simulink model "GasExample_V4S"  (R2025b)
settings: Solver=FixedStepAuto  StartTime=0.0  StopTime=1000  FixedStep=0.01  RelTol=1e-3
model workspace (MAT data in the model file):
  alpha = 20
libraries: Bibliothek_FHDO_V1 x23, BibFHDO x20, BibSpielo x11, simulink x9
(part 1 of 2)
settings Model: Creator=goessling  LastModifiedBy=henni

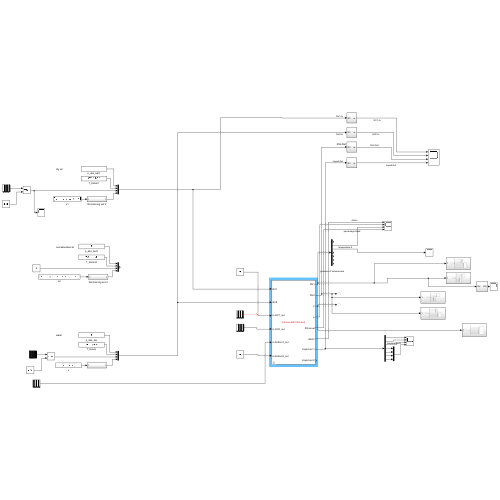
[thumbnail: Simulink's stored preview of the top-level diagram]
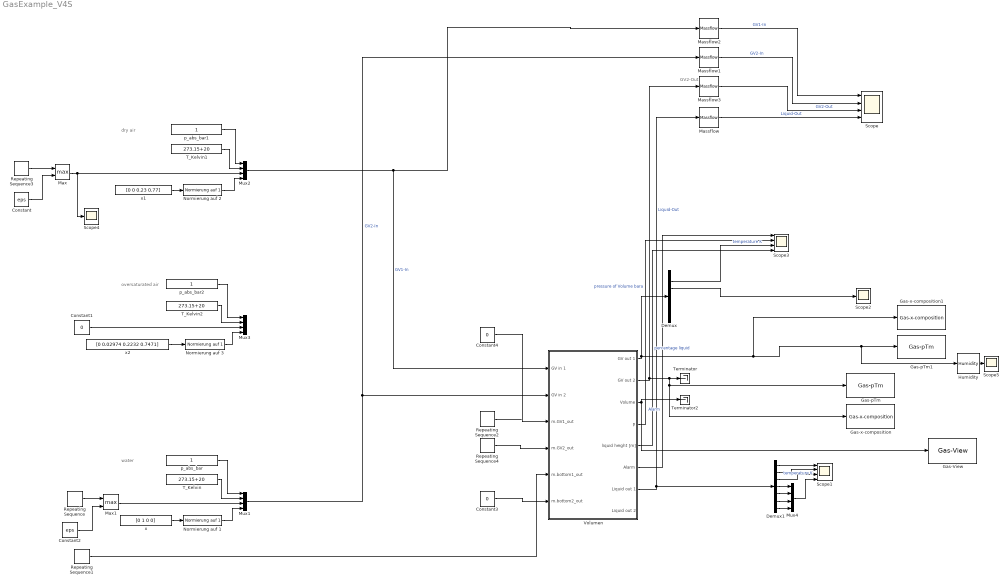
== system GasExample_V4S ==
  note: GV2-Out
  note: water
  note: dry air
  note: oversaturated air
  Constant : Constant  Value=eps
  Constant1 : Constant  Value=0
  Constant2 : Constant  Value=eps
  Constant3 : Constant  Value=0
  Constant4 : Constant  Value=0
  Demux : Demux  Outputs=7
  Demux1 : Demux  Outputs=7
  Gas-View : BibSpielo/Gas-View  SystemSampleTime=-1  VariantActivationTime=update diagram  EmptyChoice=off  PassThrough=off  PassThroughVariantControl=(default)  EmptyChoiceVariantControl=(default)  AllowFlexibleInterface=on  Latency=0  AutoFrameSizeCalculation=off
  Gas-pTm : BibSpielo/Gas-pTm  SystemSampleTime=-1  VariantActivationTime=update diagram  EmptyChoice=off  PassThrough=off  PassThroughVariantControl=(default)  EmptyChoiceVariantControl=(default)  AllowFlexibleInterface=on  Latency=0  AutoFrameSizeCalculation=off
  Gas-pTm1 : BibSpielo/Gas-pTm  SystemSampleTime=-1  VariantActivationTime=update diagram  EmptyChoice=off  PassThrough=off  PassThroughVariantControl=(default)  EmptyChoiceVariantControl=(default)  AllowFlexibleInterface=on  Latency=0  AutoFrameSizeCalculation=off
  Gas-x-composition : BibSpielo/Gas-x-composition  SystemSampleTime=-1  VariantActivationTime=update diagram  EmptyChoice=off  PassThrough=off  PassThroughVariantControl=(default)  EmptyChoiceVariantControl=(default)  AllowFlexibleInterface=on  Latency=0  AutoFrameSizeCalculation=off
  Gas-x-composition1 : BibFHDO/Gas-x-composition  SystemSampleTime=-1  VariantActivationTime=update diagram  EmptyChoice=off  PassThrough=off  PassThroughVariantControl=(default)  EmptyChoiceVariantControl=(default)  AllowFlexibleInterface=on  Latency=0  AutoFrameSizeCalculation=off
  Humidity : BibFHDO/Humidity  SystemSampleTime=-1  VariantActivationTime=update diagram  EmptyChoice=off  PassThrough=off  PassThroughVariantControl=(default)  EmptyChoiceVariantControl=(default)  AllowFlexibleInterface=on  Latency=0  AutoFrameSizeCalculation=off
  Massflow{,1..3} (4 alike) : BibSpielo/Massflow  SystemSampleTime=-1  VariantActivationTime=update diagram  EmptyChoice=off  PassThrough=off  PassThroughVariantControl=(default)  EmptyChoiceVariantControl=(default)  AllowFlexibleInterface=on  Latency=0  AutoFrameSizeCalculation=off
  Max : MinMax  Function=max  Inputs=2
  Max1 : MinMax  Function=max  Inputs=2
  Mux{1..4} (4 alike) : Mux
  Normierung auf 1 : BibSpielo/Normierung auf 1  SystemSampleTime=-1  VariantActivationTime=update diagram  EmptyChoice=off  PassThrough=off  PassThroughVariantControl=(default)  EmptyChoiceVariantControl=(default)  AllowFlexibleInterface=on  Latency=0  AutoFrameSizeCalculation=off
  Normierung auf 2 : BibSpielo/Normierung auf 1  SystemSampleTime=-1  VariantActivationTime=update diagram  EmptyChoice=off  PassThrough=off  PassThroughVariantControl=(default)  EmptyChoiceVariantControl=(default)  AllowFlexibleInterface=on  Latency=0  AutoFrameSizeCalculation=off
  Normierung auf 3 : BibSpielo/Normierung auf 1  SystemSampleTime=-1  VariantActivationTime=update diagram  EmptyChoice=off  PassThrough=off  PassThroughVariantControl=(default)  EmptyChoiceVariantControl=(default)  AllowFlexibleInterface=on  Latency=0  AutoFrameSizeCalculation=off
  Repeating Sequence : simulink/Sources/Repeating Sequence  rep_seq_t=[0 100 100.01 500 500.01 600 600.01 1000]  rep_seq_y=[1 1 0 0 1 1 0 0]*282.1778521
  Repeating Sequence1 : simulink/Sources/Repeating Sequence  rep_seq_t=[0 300 300.01 400 400.01 1000]  rep_seq_y=[0 0 1 1 0 0]*282.1778521
  Repeating Sequence2 : simulink/Sources/Repeating Sequence  rep_seq_t=[0 600 600.01 700 700.01 1000]  rep_seq_y=[0 0 1 1 0 0]*1
  Repeating Sequence3 : simulink/Sources/Repeating Sequence  rep_seq_t=[0 700 700.01 1000]  rep_seq_y=[0 0 1 1]*1
  Repeating Sequence4 : simulink/Sources/Repeating Sequence  rep_seq_t=[0 800 800.01 1000]  rep_seq_y=[0 0 1 1]*1
  Scope : Scope  NumInputPorts=4
      settings: ActiveDisplayYMinimum=-0.12499999999999972  ActiveDisplayYMaximum=1.125  DataLoggingVariableName=ScopeData5
  Scope1 : Scope  NumInputPorts=4
      settings: ActiveDisplayYMinimum=0.48520355295568851  ActiveDisplayYMaximum=7.0617394519702321
  Scope2 : Scope
      settings: ActiveDisplayYMinimum=-1.5770073931536848  ActiveDisplayYMaximum=1.2371934521588157  DataLoggingVariableName=ScopeData9
  Scope3 : Scope  NumInputPorts=4
      settings: ActiveDisplayYMinimum=-1  ActiveDisplayYMaximum=1
  Scope4 : Scope
      settings: ActiveDisplayYMinimum=-1  ActiveDisplayYMaximum=1  DataLoggingVariableName=ScopeData10
  Scope5 : Scope
      settings: ActiveDisplayYMinimum=-105.49899317481896  ActiveDisplayYMaximum=2813.8155771313386  DataLoggingVariableName=ScopeData3
  T_Kelvin : Constant  Value=273.15+20
  T_Kelvin1 : Constant  Value=273.15+20
  T_Kelvin2 : Constant  Value=273.15+20
  Terminator : Terminator
  Terminator2 : Terminator
  Volumen : Subsystem  mask{A=70685.83471/1000000, h=0.8, h_start=0.1, p_start=1, T_start=90, hum_start=50}
      mask prompts: A "Area [m^2]"; h "height [m]"; h_start "liquid level start [m]"; p_start "p [bar]"; T_start "T [°C]"; hum_start "Humidity [%]"
      mask Display:
      | color('red')
      | disp(['Volume with Fill-Level'])
      | 
      | color('black')
      | port_label('input', 1, 'GV1')
      | port_label('input', 2, 'GV2')
      | port_label('input', 3, 'm.GV1_out')
      | port_label('input', 4, 'm.GV2_out')
      | port_label('input', 5, 'm.bottom1_out')
      | port_label('input', 6, 'm.bottom2_out')
      | 
      | 
      | port_label('output', 1, 'GV1')
      | port_label('output', 2, 'GV2')
      | port_label('output', 3, 'V')
      | port_label('output', 4, 'p')
      | port_label('output', 5, 'Fill-Level')
      | port_label('output', 6, 'Alarm')
      | port_label('output', 7, 'Liquid out 1')
      | port_label('output', 8, 'Liquid out 2')
  p_abs_bar : Constant
  p_abs_bar1 : Constant
  p_abs_bar2 : Constant
  x : Constant  Value=[0 1 0 0]
  x1 : Constant  Value=[0 0 0.23 0.77]
  x2 : Constant  Value=[0 0.02974 0.2232 0.7471]
  wires:
  Volumen/3(Volume) -> Terminator2/1, Gas-View/1
  Volumen/4(p) -> Scope3/2  "pressure of Volume bara"
  Volumen/1(GV out 1) -> Gas-x-composition1/1, Humidity/1, Gas-pTm1/1, Demux/1
  Demux/2 -> Scope3/3  "temperature K"
  Volumen/5(liquid height [m]) -> Scope3/4  "percentage liquid"
  x/1 -> Normierung auf 1/1
  p_abs_bar/1 -> Mux1/1
  Mux1/1 -> Massflow1/1, Volumen/2(GV in 2)  "GV2-In"
  Repeating Sequence/1 -> Max1/1
  Normierung auf 1/1 -> Mux1/4
  T_Kelvin/1 -> Mux1/2
  T_Kelvin1/1 -> Mux2/2
  Normierung auf 2/1 -> Mux2/4
  Repeating Sequence3/1 -> Max/1
  p_abs_bar1/1 -> Mux2/1
  x1/1 -> Normierung auf 2/1
  T_Kelvin2/1 -> Mux3/2
  p_abs_bar2/1 -> Mux3/1
  x2/1 -> Normierung auf 3/1
  Normierung auf 3/1 -> Mux3/4
  Constant1/1 -> Mux3/3
  Mux2/1 -> Massflow2/1, Volumen/1(GV in 1)  "GV1-In"
  Volumen/6(Alarm) -> Scope3/1  "Alarm"
  Repeating Sequence1/1 -> Volumen/5(m.bottom1_out)
  Repeating Sequence4/1 -> Volumen/4(m.GV2_out)
  Constant3/1 -> Volumen/6(m.bottom2_out)
  Volumen/7(Liquid out 1) -> Massflow/1, Demux1/1  "Liquid-Out"
  Demux1/1 -> Scope1/1
  Demux1/2 -> Scope1/2  "temperature K"
  Demux1/3 -> Scope1/3
  Demux1/4 -> Mux4/1
  Demux1/5 -> Mux4/2
  Demux1/6 -> Mux4/3
  Demux1/7 -> Mux4/4
  Mux4/1 -> Scope1/4
  Repeating Sequence2/1 -> ?
  Constant/1 -> Max/2
  Max/1 -> Scope4/1, Mux2/3
  Constant2/1 -> Max1/2
  Max1/1 -> Mux1/3
  Constant4/1 -> Volumen/3(m.GV1_out)
  Demux/3 -> Scope2/1
  Volumen/2(GV out 2) -> Massflow3/1, Gas-pTm/1, Gas-x-composition/1, Terminator/1
  Massflow2/1 -> Scope/1  "GV1-In"
  Massflow1/1 -> Scope/2  "GV2-In"
  Massflow3/1 -> Scope/3  "GV2-Out"
  Massflow/1 -> Scope/4  "Liquid-Out"
  Humidity/1 -> Scope5/1

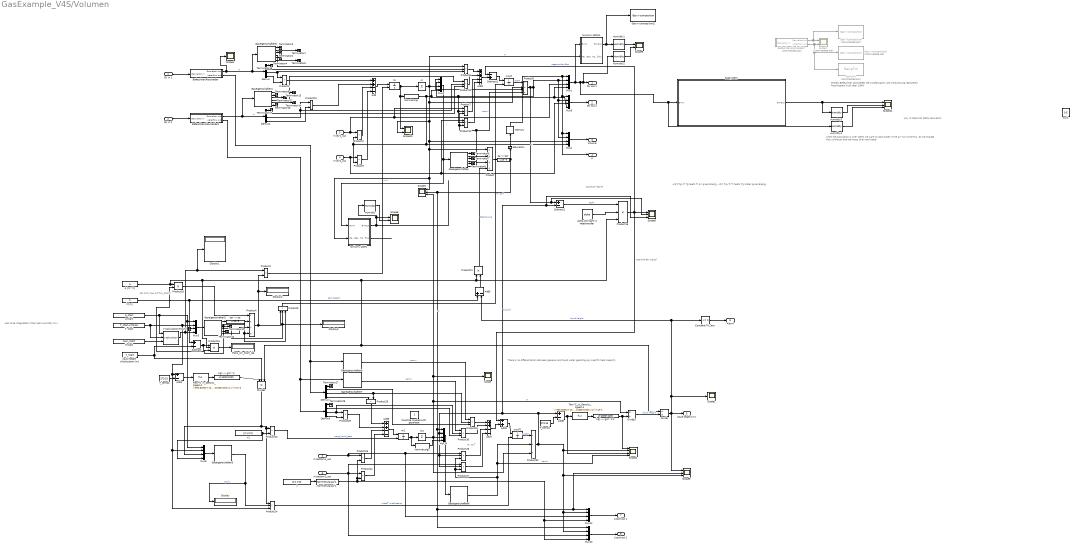
== system GasExample_V4S/Volumen ==
  note: why is there not 100% saturation
  note: when the saturation is over 100% we want to lose water in the air -[0 1 0 0]*mw.
      | So we change the x of the air and the mass of air and water
  note: Mittels Befeuchter Abscheider die Kondensation und Verdunstung realisieren
      | Feuchtigkeit nicht über 100%
  note: +Q=Tg>Tl Tg heats Tl Air gives Energy.
      | -Q= Tg<Tl Tl heats Tg Water gives Energy.
  note: 1st A*h, now A*(h-h_start)
  note: positive for Liquid
  note: Q=h*A*(Tg-Tl)
  note: There is no differentiation between gaseous and liquid water gearding e.g. spezific heat capacity
  note: m. cp T
  note: Has to be integrated in the mask Humidity to x
  GV in 1 : Inport
  GV in 2 : Inport  Port=2
  m.GV1_out : Inport  Port=3
  m.GV2_out : Inport  Port=4
  m.bottom1_out : Inport  Port=5
  m.bottom2_out : Inport  Port=6
  A [m^2] : Constant  Value=A
  Add : Sum  Inputs=++--
  Add1 : Sum  Inputs=++--  SampleTime=.01
  Add2 : Sum  Inputs=+-
  Add3 : Sum
  Add5 : Sum  Inputs=+-
  Add6 : Sum  Inputs=++--
  Add7 : Sum  Inputs=++--  SampleTime=.01
  Add8 : Sum  Inputs=+-
  Befeuchter/Abscheider : Subsystem
      mask Display:
      | color('red')
      | disp('No Oversaturation');
      | 
      | color('black')
      | port_label('output', 1, 'GV')
      | port_label('output', 2, 'm.')
      | port_label('input', 1, 'GV')
  Befeuchter/Abscheider1 : Subsystem
      mask Display:
      | color('red')
      | disp('No Oversaturation');
      | 
      | color('black')
      | port_label('output', 1, 'GV')
      | port_label('output', 2, 'm.')
      | port_label('input', 1, 'GV')
  Befeuchter/Abscheider2 : Subsystem  Commented=on
      mask Display:
      | color('red')
      | disp('No Oversaturation');
      | 
      | color('black')
      | port_label('output', 1, 'GV')
      | port_label('output', 2, 'm.')
      | port_label('input', 1, 'GV')
  Compare To Zero : simulink/Logic and Bit Operations/Compare To Zero  relop=<=  OutDataTypeStr=boolean
  Could be coupled with gasphase : Constant
  Demux{,1,4,6} (4 alike) : Demux  Outputs=[1 1 1 4]
  Display{,1..3} (4 alike) : Display
  Divide : Product  Inputs=/*
  Divide1 : Product  Inputs=*/
  Divide2 : Product  Inputs=3
  Gas-pTm : BibFHDO/Gas-pTm  Commented=on  SystemSampleTime=-1  VariantActivationTime=update diagram  EmptyChoice=off  PassThrough=off  PassThroughVariantControl=(default)  EmptyChoiceVariantControl=(default)  AllowFlexibleInterface=on  Latency=0  AutoFrameSizeCalculation=off
  Gas-x-composition : BibFHDO/Gas-x-composition  Commented=on  SystemSampleTime=-1  VariantActivationTime=update diagram  EmptyChoice=off  PassThrough=off  PassThroughVariantControl=(default)  EmptyChoiceVariantControl=(default)  AllowFlexibleInterface=on  Latency=0  AutoFrameSizeCalculation=off
  Gas-x-composition1 : BibFHDO/Gas-x-composition  Commented=on  SystemSampleTime=-1  VariantActivationTime=update diagram  EmptyChoice=off  PassThrough=off  PassThroughVariantControl=(default)  EmptyChoiceVariantControl=(default)  AllowFlexibleInterface=on  Latency=0  AutoFrameSizeCalculation=off
  Gas-x-composition2 : BibFHDO/Gas-x-composition  SystemSampleTime=-1  VariantActivationTime=update diagram  EmptyChoice=off  PassThrough=off  PassThroughVariantControl=(default)  EmptyChoiceVariantControl=(default)  AllowFlexibleInterface=on  Latency=0  AutoFrameSizeCalculation=off
  Gaseigenschaften{,1..3,5..8} (8 alike) : Bibliothek_FHDO_V1/Gaseigenschaften  SystemSampleTime=-1  VariantActivationTime=update diagram  EmptyChoice=off  PassThrough=off  PassThroughVariantControl=(default)  EmptyChoiceVariantControl=(default)  AllowFlexibleInterface=on  Latency=0  AutoFrameSizeCalculation=off
  Ground : Ground
  H start : Constant  Value=hum_start
  Humidity{,1..4} (5 alike) : BibFHDO/Humidity  SystemSampleTime=-1  VariantActivationTime=update diagram  EmptyChoice=off  PassThrough=off  PassThroughVariantControl=(default)  EmptyChoiceVariantControl=(default)  AllowFlexibleInterface=on  Latency=0  AutoFrameSizeCalculation=off
  Mass_Air_start_[g] : Display
  Memory : Memory  InitialCondition=p_start
  Mux{1..6,12..14} (9 alike) : Mux
  Normierung : Bibliothek_FHDO_V1/Sauerstoff/Normierung auf 1  SystemSampleTime=-1  VariantActivationTime=update diagram  EmptyChoice=off  PassThrough=off  PassThroughVariantControl=(default)  EmptyChoiceVariantControl=(default)  AllowFlexibleInterface=on  Latency=0  AutoFrameSizeCalculation=off
  Normierung auf 1 : Bibliothek_FHDO_V1/Wasser/Normierung auf 1  SystemSampleTime=-1  VariantActivationTime=update diagram  EmptyChoice=off  PassThrough=off  PassThroughVariantControl=(default)  EmptyChoiceVariantControl=(default)  AllowFlexibleInterface=on  Latency=0  AutoFrameSizeCalculation=off
  Normierung2 : Bibliothek_FHDO_V1/Sauerstoff/Normierung auf 1  SystemSampleTime=-1  VariantActivationTime=update diagram  EmptyChoice=off  PassThrough=off  PassThroughVariantControl=(default)  EmptyChoiceVariantControl=(default)  AllowFlexibleInterface=on  Latency=0  AutoFrameSizeCalculation=off
  Product : Product  Inputs=***/  RndMeth=Zero
  Product{1..3,9..10,13,24..25,28..29} (10 alike) : Product  RndMeth=Zero
  Product{5..7,11..12,14,26..27,30..31} (10 alike) : Product  Inputs=3  RndMeth=Zero
  Product15 : Product  Inputs=3
  Product16 : Product  Inputs=3
  Product18 : Product
  Product21 : Product
  Product32 : Product  Inputs=*//  RndMeth=Zero
  Product4 : Product  Inputs=**//  RndMeth=Zero
  Product8 : Product  Inputs=*//  RndMeth=Zero
  Saturation : Saturate  UpperLimit=inf  LowerLimit=1
  Scope : Scope
      settings: ActiveDisplayYMinimum=3528.4825816743587  ActiveDisplayYMaximum=38802.477705749261  DataLoggingVariableName=ScopeData8
  Scope1 : Scope
      settings: ActiveDisplayYMinimum=0.050007523302541844  ActiveDisplayYMaximum=0.54993229027712343  DataLoggingVariableName=ScopeData6
  Scope10 : Scope  NumInputPorts=2
      settings: ActiveDisplayYMinimum=-13.38683109586804  ActiveDisplayYMaximum=120.48147986281239  DataLoggingVariableName=ScopeData2
  Scope{3,5..6,11} (4 alike) : Scope  NumInputPorts=3
      Scope11 settings: ActiveDisplayYMinimum=-40.274654674265967  ActiveDisplayYMaximum=362.4718920683938  DataLoggingVariableName=ScopeData17
      Scope3 settings: ActiveDisplayYMinimum=60.92303202124377  ActiveDisplayYMaximum=185.9230320212491
      Scope5 settings: ActiveDisplayYMinimum=0.049993432477709931  ActiveDisplayYMaximum=0.55005910770061084  DataLoggingVariableName=ScopeData13
      Scope6 settings: ActiveDisplayYMinimum=-5.3029931830873789  ActiveDisplayYMaximum=34.215523261925469  DataLoggingVariableName=ScopeData12
  Scope2 : Scope  NumInputPorts=4
      settings: ActiveDisplayYMinimum=953445.2867554978  ActiveDisplayYMaximum=1.0024417421432E+6  DataLoggingVariableName=ScopeData7
  Scope4 : Scope
      settings: ActiveDisplayYMinimum=-0.548567099910646  ActiveDisplayYMaximum=0.95314288193326313  DataLoggingVariableName=ScopeData11
  Scope7 : Scope  Commented=on  NumInputPorts=2
      settings: ActiveDisplayYMinimum=-44.14374999999999  ActiveDisplayYMaximum=397.29375  DataLoggingVariableName=ScopeData14
  Scope8 : Scope  NumInputPorts=2
      settings: ActiveDisplayYMinimum=-37.89375  ActiveDisplayYMaximum=341.04375000000005  DataLoggingVariableName=ScopeData15
  Scope9 : Scope  NumInputPorts=2
      settings: ActiveDisplayYMinimum=33.0539149748229  ActiveDisplayYMaximum=107.41459566502954  DataLoggingVariableName=ScopeData16
  Subsystem : Subsystem
  Subtract : Sum  Inputs=+-
  Subtract1 : Sum  Inputs=+-
  Subtract2 : Sum  Inputs=-+
  T  start : Constant  Value=T_start+273.15
  T_temp1 : Constant  Value=273.15
  T_temp2 : Constant  Value=273.15
  Tem°C_in_Density_kgperL1 : Fcn  Expr=((999.83952+16.952577*u(1)-0.0079905127*u(1)^2-0.000046241757*u(1)^3+0.00000010584601*u(1)^4-0.00000000028103006*u(1)^5)/(1+0.016887236*u(1)))*1e-3
  Tem°C_in_Density_kgperL2 : Fcn  Expr=((999.83952+16.952577*u(1)-0.0079905127*u(1)^2-0.000046241757*u(1)^3+0.00000010584601*u(1)^4-0.00000000028103006*u(1)^5)/(1+0.016887236*u(1)))*1e-3
  Terminator{1..17,27..28} (19 alike) : Terminator
  alpha [W/(kg*K)] Heattransfer : Constant  Value=alpha
  "bar -> pa" : Fcn  Expr=u*10^5
  h [m] : Constant  Value=h
  "kg/l -> g/m^3" : Fcn  Expr=u*1000*1000
  "kg/l -> g/m^3 2" : Fcn  Expr=u*1000*1000
  liquid height initialization [m] : Constant  Value=h_start
  m : Sum  Inputs=+
  m2 : Sum  Inputs=+
  mcpT : Integrator  InitialConditionSource=external  InitialCondition=[0 0 0 0 0 0 .21 .79]*1293
  mcpT1 : Integrator  InitialConditionSource=external  InitialCondition=[0 0 0 0 0 0 .21 .79]*1293
  mi : Integrator  InitialConditionSource=external  InitialCondition=[0 0 0 0 0 0 .21 .79]*1293
  mi1 : Integrator  InitialConditionSource=external  InitialCondition=[0 0 0 0 0 0 .21 .79]*1293
  mwk. : Constant  Value=0.5
  no Hum>100% : Subsystem
  no Hum>100%1 : Subsystem
  p start : Constant  Value=p_start
  "pa -> bar" : Fcn  Expr=u/10^5
  x : Constant  Value=[0 1 0 0]
  x-Calculation : BibFHDO/x-Calculation  SystemSampleTime=-1  VariantActivationTime=update diagram  EmptyChoice=off  PassThrough=off  PassThroughVariantControl=(default)  EmptyChoiceVariantControl=(default)  AllowFlexibleInterface=on  Latency=0  AutoFrameSizeCalculation=off
  x1 : Constant  Value=[0 1 0 0]
  GV out 1 : Outport
  GV out 2 : Outport  Port=2
  Volume : Outport  Port=3
  p : Outport  Port=4
  liquid height [m] : Outport  Port=5
  Alarm : Outport  Port=6
  Liquid out 1 : Outport  Port=7
  Liquid out 2 : Outport  Port=8
  wires:
  GV in 1/1 -> Befeuchter/Abscheider/1(Gasvektor in)
  Demux/3 -> Product1/1, Product6/3
  Demux/2 -> Product6/2
  Demux/4 -> Product1/2
  Gaseigenschaften/1 -> Terminator6/1
  Gaseigenschaften/4 -> Product8/3, Product7/3, Product12/3  "cpmix"
  Product1/1 -> Add/1
  m.GV1_out/1 -> Product2/1, Product7/1, Mux1/3
  Normierung/1 -> Mux2/4, Mux1/4, Mux5/4, Mux4/4, Product9/2, Product2/2
  Product2/1 -> Add/3
  Add/1 -> mi/1
  m/1 -> Scope3/1, no Hum>100%/2(Mass-Gas), Product/1, Mux4/3, Scope10/2, Product8/2, no Hum>100%1/2(Mass-Gas), Mux2/3  "m"
  Gaseigenschaften5/1 -> Terminator3/1
  Gaseigenschaften/6 -> Product/3
  Gaseigenschaften/2 -> Product/2
  A [m^2]/1 -> Product15/2, Divide2/3, Divide/1, Product16/3, Product21/1, Product18/1
  Product/1 -> "pa -> bar"/1
  Gaseigenschaften5/2 -> Terminator1/1
  Gaseigenschaften5/3 -> Terminator2/1
  Gaseigenschaften5/5 -> Terminator4/1
  Gaseigenschaften5/6 -> Terminator5/1
  Gaseigenschaften/3 -> Terminator7/1
  Gaseigenschaften/5 -> Terminator8/1
  Ground/1 -> Mux3/3
  p start/1 -> x-Calculation/1, Mux3/1, Mux6/1
  T  start/1 -> x-Calculation/2, Mux6/2, Product14/3, Add2/1, Mux3/2
  Mux3/1 -> Gaseigenschaften2/1
  Gaseigenschaften2/1 -> "bar -> pa"/1
  "bar -> pa"/1 -> Product4/2
  Gaseigenschaften2/6 -> Product4/3
  Gaseigenschaften2/2 -> Product4/4, Product5/3
  Gaseigenschaften2/3 -> Product15/3, Terminator11/1
  Gaseigenschaften2/4 -> Display3/1, Product5/2
  Gaseigenschaften2/5 -> Terminator10/1
  Product4/1 -> Display2/1, Product3/2, Product5/1
  Product3/1 -> mi/2  "m*x"
  Product5/1 -> mcpT/2  "m. cp T"
  Product6/1 -> Add1/1
  mcpT/1 -> Product8/1  "mcpT"
  Product8/1 -> Scope6/2, Subtract1/1, Mux2/2, Product7/2, Product12/2, Mux1/2, Mux5/2, Mux4/2  "T"
  Product7/1 -> Add1/3
  m.GV2_out/1 -> Product9/1, Mux5/3, Product12/1
  Product9/1 -> Add/4
  Mux5/1 -> GV out 2/1
  Gaseigenschaften1/1 -> Terminator13/1
  Gaseigenschaften1/2 -> Terminator9/1
  Gaseigenschaften1/3 -> Terminator12/1
  Gaseigenschaften1/5 -> Terminator14/1
  Gaseigenschaften1/6 -> Terminator15/1
  Demux/1 -> Terminator16/1
  Demux1/1 -> Terminator17/1
  Demux1/3 -> Product11/2, Product10/1
  Demux1/4 -> Product10/2
  Product10/1 -> Add/2
  Product11/1 -> Add1/2
  Product12/1 -> Add1/4
  Gaseigenschaften1/4 -> Product11/1
  Demux1/2 -> Product11/3
  Saturation/1 -> Memory/1
  Mux4/1 -> Volume/1
  mi/1 -> Scope10/1, Normierung/1, m/1
  h [m]/1 -> Add5/1, Subtract/1  "tank height"
  Add5/1 -> Product21/2
  Product21/1 -> Product/4  "GasVolume"
  Product18/1 -> Product4/1
  "pa -> bar"/1 -> Saturation/1, Scope5/2, Mux12/1, Mux13/1, Mux14/1, Scope3/2  "p"
  Mux2/1 -> Gaseigenschaften/1, no Hum>100%/1(GV-In)
  x/1 -> Normierung auf 1/1
  Normierung auf 1/1 -> Mux13/4, Mux12/4, Product25/2, Product24/2
  m.bottom2_out/1 -> Product27/1, Product24/1, Mux13/3
  m.bottom1_out/1 -> Product25/1, Mux12/3, Product26/1
  Mux12/1 -> Liquid out 1/1
  Mux13/1 -> Liquid out 2/1
  Product25/1 -> Add6/3
  Product24/1 -> Add6/4
  Befeuchter/Abscheider/1(Gasvektor out) -> Scope4/1, Demux/1, Gaseigenschaften5/1  "m"
  GV in 2/1 -> Befeuchter/Abscheider1/1(Gasvektor in)
  Befeuchter/Abscheider1/1(Gasvektor out) -> Gaseigenschaften1/1, Demux1/1  "m"
  Befeuchter/Abscheider/2(waterflow out) -> Demux4/1, Gaseigenschaften8/1
  Befeuchter/Abscheider1/2(waterflow out) -> Demux6/1, Gaseigenschaften7/1
  Demux4/4 -> Product28/1
  Demux4/1 -> Terminator27/1
  Demux4/3 -> Product31/2, Product28/2
  Demux6/3 -> Product30/2, Product29/1
  Demux6/1 -> Terminator28/1
  Demux6/4 -> Product29/2
  Product28/1 -> Add6/1
  Product29/1 -> Add6/2
  Add6/1 -> mi1/1
  mi1/1 -> Normierung2/1, m2/1
  m2/1 -> Scope3/3, Scope/1, Divide1/1, Product32/3, Mux14/3  "m"
  Product32/1 -> Scope6/3, Subtract1/2, Product27/2, Product26/2, Mux14/2, Add8/1, Scope5/3, Mux12/2, Mux13/2, Scope2/2  "TLiquid"
  Normierung2/1 -> Mux14/4
  Mux14/1 -> Gaseigenschaften6/1
  Gaseigenschaften8/4 -> Product31/1  "cpmix"
  Gaseigenschaften7/4 -> Product30/1  "cpmix"
  Demux4/2 -> Product31/3
  Demux6/2 -> Product30/3
  Product31/1 -> Add7/1
  Product30/1 -> Add7/2
  Gaseigenschaften6/4 -> Product27/3, Product26/3, Scope2/4, Product32/2  "cpmix"
  Product26/1 -> Add7/3
  Product27/1 -> Add7/4
  Add7/1 -> Add3/2
  mcpT1/1 -> Product32/1  "mcpT"
  Tem°C_in_Density_kgperL1/1 -> "kg/l -> g/m^3 2"/1
  T_temp1/1 -> Add8/2
  Add8/1 -> Scope2/3, Tem°C_in_Density_kgperL1/1
  "kg/l -> g/m^3 2"/1 -> Scope2/1, Divide1/2
  Divide/1 -> liquid height [m]/1, Scope1/1, Compare To Zero/1, Add5/2, Scope5/1  "liquid height"
  Divide1/1 -> Divide/2  "liquid height"
  Divide2/1 -> Product14/1, Product13/1, Mux6/3
  Memory/1 -> Mux5/1, p/1, Mux4/1, Mux1/1, Mux2/1
  Compare To Zero/1 -> Alarm/1
  Add2/1 -> Tem°C_in_Density_kgperL2/1
  T_temp2/1 -> Add2/2
  Tem°C_in_Density_kgperL2/1 -> "kg/l -> g/m^3"/1
  liquid height initialization [m]/1 -> Subtract/2, Divide2/2
  x1/1 -> Product13/2, Mux6/4
  Product13/1 -> mi1/2  "mass_liquid_start"
  Mux6/1 -> Gaseigenschaften3/1
  Gaseigenschaften3/4 -> Display/1, Product14/2  "cpmix"
  Product14/1 -> mcpT1/2  "mcpdT initialization"
  Gaseigenschaften5/4 -> Product6/1
  "kg/l -> g/m^3"/1 -> Divide2/1
  x-Calculation/1 -> Display1/1, Product3/1, Mux3/4
  H start/1 -> x-Calculation/3
  Product15/1 -> Mass_Air_start_[g]/1
  Subtract1/1 -> Product16/1  "Tg-Tl"
  alpha [W/(kg*K)] Heattransfer/1 -> Product16/2
  Product16/1 -> Subtract2/1, Scope6/1, Add3/1  "negative for Gas"
  Add1/1 -> Subtract2/2
  Subtract2/1 -> mcpT/1
  Add3/1 -> mcpT1/1
  Subtract/1 -> Product18/2, Product15/1
  Befeuchter/Abscheider2/1(Gasvektor out) -> Gas-x-composition/1, Scope7/1
  Befeuchter/Abscheider2/2(waterflow out) -> Gas-pTm/1, Gas-x-composition1/1, Scope7/2
  no Hum>100%/2(H2O-flow) -> ?
  Humidity/1 -> Scope8/2
  no Hum>100%/1(GV-Out) -> Humidity/1, Scope8/1
  no Hum>100%1/1(GV-Out) -> Gas-x-composition2/1, Humidity1/1
  Humidity1/1 -> Scope9/1
  Humidity2/1 -> Scope9/2
  Mux1/1 -> no Hum>100%1/1(GV-In), Humidity4/1, Subsystem/1(GV-In), Humidity2/1, GV out 1/1
  Subsystem/1(GV-Out) -> Humidity3/1, Scope11/1
  Humidity3/1 -> Scope11/2
  Humidity4/1 -> Scope11/3

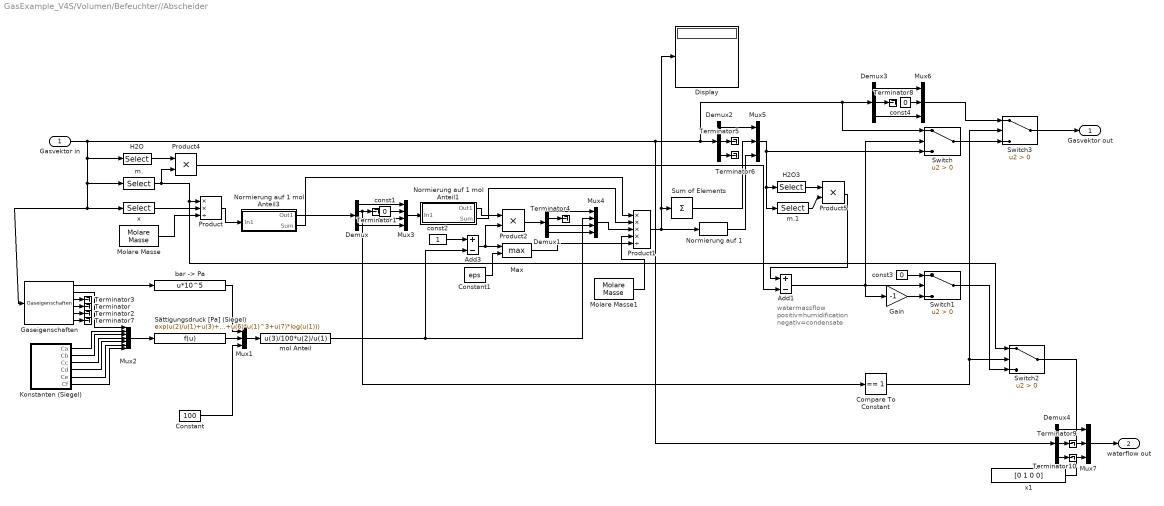
== system GasExample_V4S/Volumen/Befeuchter//Abscheider ==
  note: watermassflow
      | positiv=humidification
      | negativ=condensate
  Gasvektor in : Inport
  Add1 : Sum  Inputs=+-
  Add3 : Sum  Inputs=+-
  Compare To Constant : simulink/Logic and Bit Operations/Compare To Constant  relop===  const=1  OutDataTypeStr=boolean
  Constant : Constant  Value=100
  Constant1 : Constant  Value=eps
  Demux : Demux
  Demux1 : Demux
  Demux2 : Demux  Outputs=[2 1 4]
  Demux3 : Demux  Outputs=[2 1 4]
  Demux4 : Demux  Outputs=[2 1 4]
  Display : Display
  Gain : Gain  Gain=-1
  Gaseigenschaften : Bibliothek_FHDO_V1/Gaseigenschaften  SystemSampleTime=-1  VariantActivationTime=update diagram  EmptyChoice=off  PassThrough=off  PassThroughVariantControl=(default)  EmptyChoiceVariantControl=(default)  AllowFlexibleInterface=on  Latency=0  AutoFrameSizeCalculation=off
  H2O : Selector  InputPortWidth=7  IndexOptions=Index vector (dialog)  Indices=5  OutputSizes=1
  H2O3 : Selector  InputPortWidth=7  IndexOptions=Index vector (dialog)  Indices=5  OutputSizes=1
  Konstanten (Siegel) : Subsystem
  Max : MinMax  Function=max  Inputs=2
  Molare Masse : Bibliothek_FHDO_V1/Molare Masse  SystemSampleTime=-1  VariantActivationTime=update diagram  EmptyChoice=off  PassThrough=off  PassThroughVariantControl=(default)  EmptyChoiceVariantControl=(default)  AllowFlexibleInterface=on  Latency=0  AutoFrameSizeCalculation=off
  Molare Masse1 : Bibliothek_FHDO_V1/Molare Masse  SystemSampleTime=-1  VariantActivationTime=update diagram  EmptyChoice=off  PassThrough=off  PassThroughVariantControl=(default)  EmptyChoiceVariantControl=(default)  AllowFlexibleInterface=on  Latency=0  AutoFrameSizeCalculation=off
  Mux{1,5..7} (4 alike) : Mux  Inputs=3
  Mux2 : Mux  Inputs=7
  Mux3 : Mux
  Mux4 : Mux
  Normierung auf 1 : Bibliothek_FHDO_V1/Sauerstoff/Normierung auf 1  SystemSampleTime=-1  VariantActivationTime=update diagram  EmptyChoice=off  PassThrough=off  PassThroughVariantControl=(default)  EmptyChoiceVariantControl=(default)  AllowFlexibleInterface=on  Latency=0  AutoFrameSizeCalculation=off
  Normierung auf 1 mol Anteil1 : Subsystem
  Normierung auf 1 mol Anteil3 : Subsystem
  Product : Product  Inputs=**/  RndMeth=Zero
  Product1 : Product  Inputs=****/  RndMeth=Zero
  Product2 : Product  RndMeth=Zero
  Product4 : Product  RndMeth=Zero
  Product5 : Product  RndMeth=Zero
  Sum of Elements : Sum  Inputs=+
  Switch{,1..3} (4 alike) : Switch  Criteria=u2 > Threshold  SaturateOnIntegerOverflow=off  InputSameDT=off
  Sättigungsdruck [Pa] (Siegel) : Fcn  Expr=exp(u(2)/u(1)+u(3)+u(4)*u(1)+u(5)*u(1)^2+u(6)*u(1)^3+u(7)*log(u(1)))
  Terminator{,1..10} (11 alike) : Terminator
  "bar -> Pa" : Fcn  Expr=u*10^5
  const1 : Constant  Value=0
  const2 : Constant
  const3 : Constant  Value=0
  const4 : Constant  Value=0
  m. : Selector  InputPortWidth=7  IndexOptions=Index vector (dialog)  Indices=3  OutputSizes=1
  m.1 : Selector  InputPortWidth=7  IndexOptions=Index vector (dialog)  Indices=3  OutputSizes=1
  mol Anteil : Fcn  Expr=u(3)/100*u(2)/u(1)
  x : Selector  InputPortWidth=7  IndexOptions=Index vector (dialog)  Indices=[4 5 6 7]  OutputSizes=1
  x1 : Constant  Value=[0 1 0 0]
  Gasvektor out : Outport
  waterflow out : Outport  Port=2
  wires:
  Demux1/4 -> Mux4/4
  Demux1/3 -> Mux4/3
  Demux1/1 -> Mux4/1
  Demux1/2 -> Terminator4/1
  Demux/4 -> Mux3/4
  Demux/3 -> Mux3/3
  Demux/1 -> Mux3/1
  const1/1 -> Mux3/2
  Demux/2 -> Compare To Constant/1, Terminator1/1
  Product4/1 -> Add1/2
  Product5/1 -> Add1/1
  H2O3/1 -> Product5/1
  m.1/1 -> Product5/2
  H2O/1 -> Product4/1
  Normierung auf 1 mol Anteil1/2(Sum) -> Product1/2
  Normierung auf 1 mol Anteil3/2(Sum) -> Product1/1
  Normierung auf 1 mol Anteil3/1(Out1) -> Demux/1
  Normierung auf 1/1 -> Mux5/3
  Mux5/1 -> Switch/3, m.1/1, H2O3/1
  Demux2/3 -> Terminator6/1
  Demux2/2 -> Terminator5/1
  Product1/1 -> Normierung auf 1/1, Display/1, Sum of Elements/1
  Sum of Elements/1 -> Mux5/2
  Demux2/1 -> Mux5/1
  m./1 -> Switch2/1, Product/1, Product4/2
  Molare Masse1/1 -> Product1/4
  Mux4/1 -> Product1/3
  Product2/1 -> Demux1/1
  Add3/1 -> Max/1, Product2/2
  Normierung auf 1 mol Anteil1/1(Out1) -> Product2/1
  mol Anteil/1 -> Mux4/2, Add3/2
  const2/1 -> Add3/1
  Mux3/1 -> Normierung auf 1 mol Anteil1/1(In1)
  Product/1 -> Normierung auf 1 mol Anteil3/1(In1)
  Molare Masse/1 -> Product/3
  x/1 -> Product/2
  "bar -> Pa"/1 -> Mux1/1
  Constant/1 -> Mux1/3
  Mux1/1 -> mol Anteil/1
  Sättigungsdruck [Pa] (Siegel)/1 -> Mux1/2
  Mux2/1 -> Sättigungsdruck [Pa] (Siegel)/1
  Gaseigenschaften/5 -> Terminator2/1
  Gaseigenschaften/4 -> Terminator/1
  Gaseigenschaften/3 -> Terminator3/1
  Gaseigenschaften/1 -> "bar -> Pa"/1
  Konstanten (Siegel)/6(Cf) -> Mux2/7
  Konstanten (Siegel)/5(Ce) -> Mux2/6
  Konstanten (Siegel)/4(Cd) -> Mux2/5
  Konstanten (Siegel)/3(Cc) -> Mux2/4
  Konstanten (Siegel)/2(Cb) -> Mux2/3
  Konstanten (Siegel)/1(Ca) -> Mux2/2
  Gaseigenschaften/2 -> Mux2/1
  Gasvektor in/1 -> Switch/1, Demux3/1, Demux2/1, Demux4/1, H2O/1, Gaseigenschaften/1, x/1, m./1
  Gaseigenschaften/6 -> Terminator7/1
  Add1/1 -> Gain/1, Switch1/2, Switch/2
  Switch/1 -> Switch3/3
  const3/1 -> Switch1/1
  Compare To Constant/1 -> Switch3/2, Switch2/2
  Switch2/1 -> Mux7/2
  Switch1/1 -> Switch2/3
  Demux3/1 -> Mux6/1
  Demux3/3 -> Mux6/3
  const4/1 -> Mux6/2
  Demux3/2 -> Terminator8/1
  Mux6/1 -> Switch3/1
  Switch3/1 -> Gasvektor out/1
  Demux4/1 -> Mux7/1
  Demux4/2 -> Terminator9/1
  Demux4/3 -> Terminator10/1
  x1/1 -> Mux7/3
  Mux7/1 -> waterflow out/1
  Gain/1 -> Switch1/3
  Constant1/1 -> Max/2
  Max/1 -> Product1/5

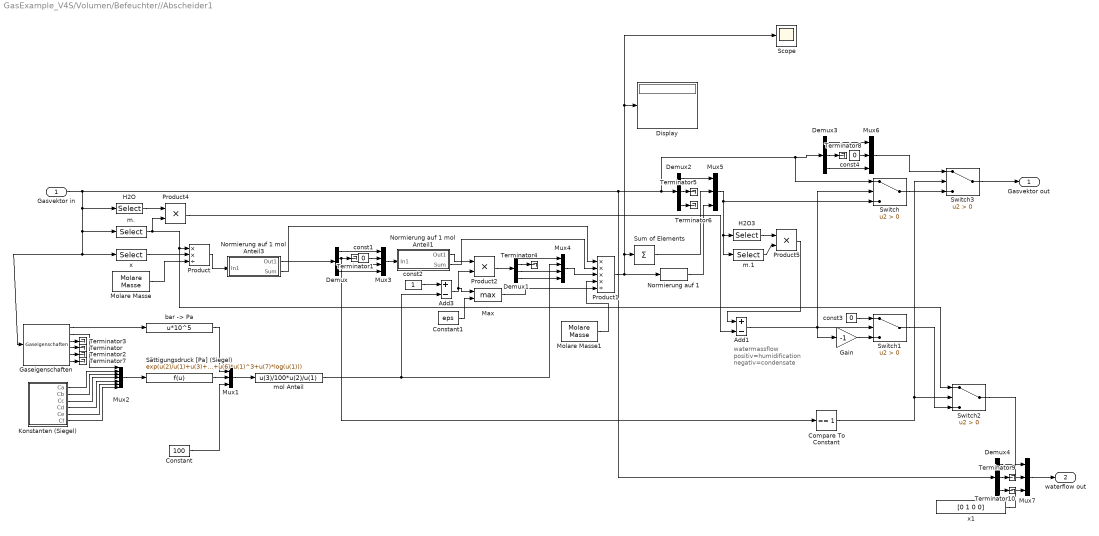
== system GasExample_V4S/Volumen/Befeuchter//Abscheider1 ==
  note: watermassflow
      | positiv=humidification
      | negativ=condensate
  Gasvektor in : Inport
  Add1 : Sum  Inputs=+-
  Add3 : Sum  Inputs=+-
  Compare To Constant : simulink/Logic and Bit Operations/Compare To Constant  relop===  const=1  OutDataTypeStr=boolean
  Constant : Constant  Value=100
  Constant1 : Constant  Value=eps
  Demux : Demux
  Demux1 : Demux
  Demux2 : Demux  Outputs=[2 1 4]
  Demux3 : Demux  Outputs=[2 1 4]
  Demux4 : Demux  Outputs=[2 1 4]
  Display : Display
  Gain : Gain  Gain=-1
  Gaseigenschaften : Bibliothek_FHDO_V1/Gaseigenschaften  SystemSampleTime=-1  VariantActivationTime=update diagram  EmptyChoice=off  PassThrough=off  PassThroughVariantControl=(default)  EmptyChoiceVariantControl=(default)  AllowFlexibleInterface=on  Latency=0  AutoFrameSizeCalculation=off
  H2O : Selector  InputPortWidth=7  IndexOptions=Index vector (dialog)  Indices=5  OutputSizes=1
  H2O3 : Selector  InputPortWidth=7  IndexOptions=Index vector (dialog)  Indices=5  OutputSizes=1
  Konstanten (Siegel) : Subsystem
  Max : MinMax  Function=max  Inputs=2
  Molare Masse : Bibliothek_FHDO_V1/Molare Masse  SystemSampleTime=-1  VariantActivationTime=update diagram  EmptyChoice=off  PassThrough=off  PassThroughVariantControl=(default)  EmptyChoiceVariantControl=(default)  AllowFlexibleInterface=on  Latency=0  AutoFrameSizeCalculation=off
  Molare Masse1 : Bibliothek_FHDO_V1/Molare Masse  SystemSampleTime=-1  VariantActivationTime=update diagram  EmptyChoice=off  PassThrough=off  PassThroughVariantControl=(default)  EmptyChoiceVariantControl=(default)  AllowFlexibleInterface=on  Latency=0  AutoFrameSizeCalculation=off
  Mux{1,5..7} (4 alike) : Mux  Inputs=3
  Mux2 : Mux  Inputs=7
  Mux3 : Mux
  Mux4 : Mux
  Normierung auf 1 : Bibliothek_FHDO_V1/Sauerstoff/Normierung auf 1  SystemSampleTime=-1  VariantActivationTime=update diagram  EmptyChoice=off  PassThrough=off  PassThroughVariantControl=(default)  EmptyChoiceVariantControl=(default)  AllowFlexibleInterface=on  Latency=0  AutoFrameSizeCalculation=off
  Normierung auf 1 mol Anteil1 : Subsystem
  Normierung auf 1 mol Anteil3 : Subsystem
  Product : Product  Inputs=**/  RndMeth=Zero
  Product1 : Product  Inputs=****/  RndMeth=Zero
  Product2 : Product  RndMeth=Zero
  Product4 : Product  RndMeth=Zero
  Product5 : Product  RndMeth=Zero
  Scope : Scope
      settings: ActiveDisplayYMinimum=-0.33566791747822972  ActiveDisplayYMaximum=0.418111048267771  DataLoggingVariableName=ScopeData4
  Sum of Elements : Sum  Inputs=+
  Switch{,1..3} (4 alike) : Switch  Criteria=u2 > Threshold  SaturateOnIntegerOverflow=off  InputSameDT=off
  Sättigungsdruck [Pa] (Siegel) : Fcn  Expr=exp(u(2)/u(1)+u(3)+u(4)*u(1)+u(5)*u(1)^2+u(6)*u(1)^3+u(7)*log(u(1)))
  Terminator{,1..10} (11 alike) : Terminator
  "bar -> Pa" : Fcn  Expr=u*10^5
  const1 : Constant  Value=0
  const2 : Constant
  const3 : Constant  Value=0
  const4 : Constant  Value=0
  m. : Selector  InputPortWidth=7  IndexOptions=Index vector (dialog)  Indices=3  OutputSizes=1
  m.1 : Selector  InputPortWidth=7  IndexOptions=Index vector (dialog)  Indices=3  OutputSizes=1
  mol Anteil : Fcn  Expr=u(3)/100*u(2)/u(1)
  x : Selector  InputPortWidth=7  IndexOptions=Index vector (dialog)  Indices=[4 5 6 7]  OutputSizes=1
  x1 : Constant  Value=[0 1 0 0]
  Gasvektor out : Outport
  waterflow out : Outport  Port=2
  wires:
  Max/1 -> Product1/5
  Constant1/1 -> Max/2
  Gain/1 -> Switch1/3
  Mux7/1 -> waterflow out/1
  x1/1 -> Mux7/3
  Demux4/3 -> Terminator10/1
  Demux4/2 -> Terminator9/1
  Demux4/1 -> Mux7/1
  Switch3/1 -> Gasvektor out/1
  Mux6/1 -> Switch3/1
  Demux3/2 -> Terminator8/1
  const4/1 -> Mux6/2
  Demux3/3 -> Mux6/3
  Demux3/1 -> Mux6/1
  Switch1/1 -> Switch2/3
  Switch2/1 -> Mux7/2
  Compare To Constant/1 -> Switch2/2, Switch3/2
  const3/1 -> Switch1/1
  Switch/1 -> Switch3/3
  Add1/1 -> Switch/2, Switch1/2, Gain/1
  Gaseigenschaften/6 -> Terminator7/1
  Gasvektor in/1 -> m./1, x/1, Gaseigenschaften/1, H2O/1, Demux4/1, Demux2/1, Switch/1, Demux3/1
  Gaseigenschaften/2 -> Mux2/1
  Konstanten (Siegel)/1(Ca) -> Mux2/2
  Konstanten (Siegel)/2(Cb) -> Mux2/3
  Konstanten (Siegel)/3(Cc) -> Mux2/4
  Konstanten (Siegel)/4(Cd) -> Mux2/5
  Konstanten (Siegel)/5(Ce) -> Mux2/6
  Konstanten (Siegel)/6(Cf) -> Mux2/7
  Gaseigenschaften/1 -> "bar -> Pa"/1
  Gaseigenschaften/3 -> Terminator3/1
  Gaseigenschaften/4 -> Terminator/1
  Gaseigenschaften/5 -> Terminator2/1
  Mux2/1 -> Sättigungsdruck [Pa] (Siegel)/1
  Sättigungsdruck [Pa] (Siegel)/1 -> Mux1/2
  Mux1/1 -> mol Anteil/1
  Constant/1 -> Mux1/3
  "bar -> Pa"/1 -> Mux1/1
  x/1 -> Product/2
  Molare Masse/1 -> Product/3
  Product/1 -> Normierung auf 1 mol Anteil3/1(In1)
  Mux3/1 -> Normierung auf 1 mol Anteil1/1(In1)
  const2/1 -> Add3/1
  mol Anteil/1 -> Add3/2, Mux4/2
  Normierung auf 1 mol Anteil1/1(Out1) -> Product2/1
  Add3/1 -> Product2/2, Max/1
  Product2/1 -> Demux1/1
  Mux4/1 -> Product1/3
  Molare Masse1/1 -> Product1/4
  m./1 -> Product4/2, Product/1, Switch2/1
  Demux2/1 -> Mux5/1
  Sum of Elements/1 -> Mux5/2
  Product1/1 -> Sum of Elements/1, Scope/1, Display/1, Normierung auf 1/1
  Demux2/2 -> Terminator5/1
  Demux2/3 -> Terminator6/1
  Mux5/1 -> H2O3/1, m.1/1, Switch/3
  Normierung auf 1/1 -> Mux5/3
  Normierung auf 1 mol Anteil3/1(Out1) -> Demux/1
  Normierung auf 1 mol Anteil3/2(Sum) -> Product1/1
  Normierung auf 1 mol Anteil1/2(Sum) -> Product1/2
  H2O/1 -> Product4/1
  m.1/1 -> Product5/2
  H2O3/1 -> Product5/1
  Product5/1 -> Add1/1
  Product4/1 -> Add1/2
  Demux/2 -> Terminator1/1, Compare To Constant/1
  const1/1 -> Mux3/2
  Demux/1 -> Mux3/1
  Demux/3 -> Mux3/3
  Demux/4 -> Mux3/4
  Demux1/2 -> Terminator4/1
  Demux1/1 -> Mux4/1
  Demux1/3 -> Mux4/3
  Demux1/4 -> Mux4/4

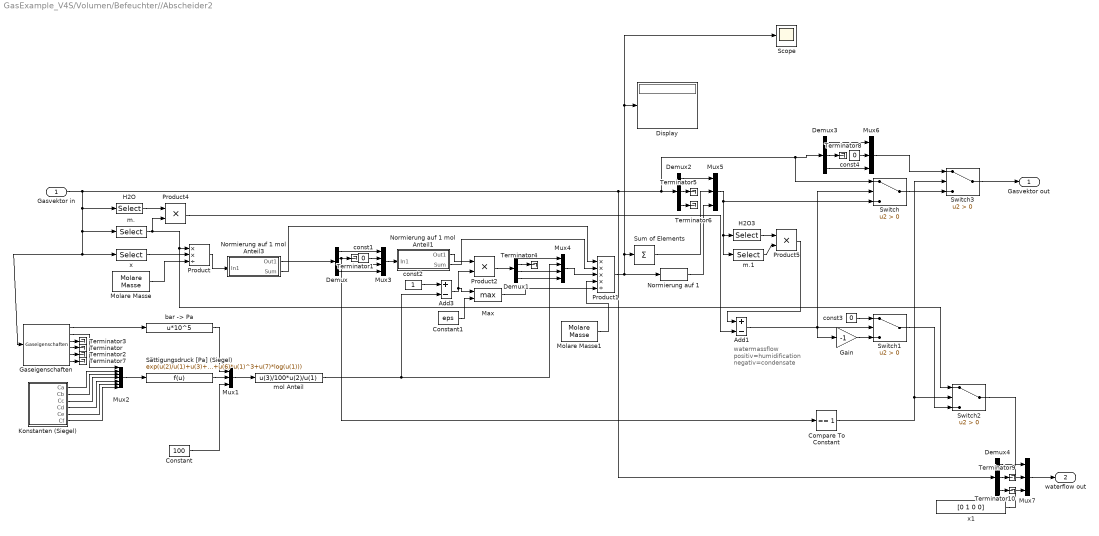
== system GasExample_V4S/Volumen/Befeuchter//Abscheider2 ==
  note: watermassflow
      | positiv=humidification
      | negativ=condensate
  Gasvektor in : Inport
  Add1 : Sum  Inputs=+-
  Add3 : Sum  Inputs=+-
  Compare To Constant : simulink/Logic and Bit Operations/Compare To Constant  relop===  const=1  OutDataTypeStr=boolean
  Constant : Constant  Value=100
  Constant1 : Constant  Value=eps
  Demux : Demux
  Demux1 : Demux
  Demux2 : Demux  Outputs=[2 1 4]
  Demux3 : Demux  Outputs=[2 1 4]
  Demux4 : Demux  Outputs=[2 1 4]
  Display : Display
  Gain : Gain  Gain=-1
  Gaseigenschaften : Bibliothek_FHDO_V1/Gaseigenschaften  SystemSampleTime=-1  VariantActivationTime=update diagram  EmptyChoice=off  PassThrough=off  PassThroughVariantControl=(default)  EmptyChoiceVariantControl=(default)  AllowFlexibleInterface=on  Latency=0  AutoFrameSizeCalculation=off
  H2O : Selector  InputPortWidth=7  IndexOptions=Index vector (dialog)  Indices=5  OutputSizes=1
  H2O3 : Selector  InputPortWidth=7  IndexOptions=Index vector (dialog)  Indices=5  OutputSizes=1
  Konstanten (Siegel) : Subsystem
  Max : MinMax  Function=max  Inputs=2
  Molare Masse : Bibliothek_FHDO_V1/Molare Masse  SystemSampleTime=-1  VariantActivationTime=update diagram  EmptyChoice=off  PassThrough=off  PassThroughVariantControl=(default)  EmptyChoiceVariantControl=(default)  AllowFlexibleInterface=on  Latency=0  AutoFrameSizeCalculation=off
  Molare Masse1 : Bibliothek_FHDO_V1/Molare Masse  SystemSampleTime=-1  VariantActivationTime=update diagram  EmptyChoice=off  PassThrough=off  PassThroughVariantControl=(default)  EmptyChoiceVariantControl=(default)  AllowFlexibleInterface=on  Latency=0  AutoFrameSizeCalculation=off
  Mux{1,5..7} (4 alike) : Mux  Inputs=3
  Mux2 : Mux  Inputs=7
  Mux3 : Mux
  Mux4 : Mux
  Normierung auf 1 : Bibliothek_FHDO_V1/Sauerstoff/Normierung auf 1  SystemSampleTime=-1  VariantActivationTime=update diagram  EmptyChoice=off  PassThrough=off  PassThroughVariantControl=(default)  EmptyChoiceVariantControl=(default)  AllowFlexibleInterface=on  Latency=0  AutoFrameSizeCalculation=off
  Normierung auf 1 mol Anteil1 : Subsystem
  Normierung auf 1 mol Anteil3 : Subsystem
  Product : Product  Inputs=**/  RndMeth=Zero
  Product1 : Product  Inputs=****/  RndMeth=Zero
  Product2 : Product  RndMeth=Zero
  Product4 : Product  RndMeth=Zero
  Product5 : Product  RndMeth=Zero
  Scope : Scope
      settings: ActiveDisplayYMinimum=-0.33566791747822972  ActiveDisplayYMaximum=0.418111048267771  DataLoggingVariableName=ScopeData4
  Sum of Elements : Sum  Inputs=+
  Switch{,1..3} (4 alike) : Switch  Criteria=u2 > Threshold  SaturateOnIntegerOverflow=off  InputSameDT=off
  Sättigungsdruck [Pa] (Siegel) : Fcn  Expr=exp(u(2)/u(1)+u(3)+u(4)*u(1)+u(5)*u(1)^2+u(6)*u(1)^3+u(7)*log(u(1)))
  Terminator{,1..10} (11 alike) : Terminator
  "bar -> Pa" : Fcn  Expr=u*10^5
  const1 : Constant  Value=0
  const2 : Constant
  const3 : Constant  Value=0
  const4 : Constant  Value=0
  m. : Selector  InputPortWidth=7  IndexOptions=Index vector (dialog)  Indices=3  OutputSizes=1
  m.1 : Selector  InputPortWidth=7  IndexOptions=Index vector (dialog)  Indices=3  OutputSizes=1
  mol Anteil : Fcn  Expr=u(3)/100*u(2)/u(1)
  x : Selector  InputPortWidth=7  IndexOptions=Index vector (dialog)  Indices=[4 5 6 7]  OutputSizes=1
  x1 : Constant  Value=[0 1 0 0]
  Gasvektor out : Outport
  waterflow out : Outport  Port=2
  wires:
  Demux1/4 -> Mux4/4
  Demux1/3 -> Mux4/3
  Demux1/1 -> Mux4/1
  Demux1/2 -> Terminator4/1
  Demux/4 -> Mux3/4
  Demux/3 -> Mux3/3
  Demux/1 -> Mux3/1
  const1/1 -> Mux3/2
  Demux/2 -> Compare To Constant/1, Terminator1/1
  Product4/1 -> Add1/2
  Product5/1 -> Add1/1
  H2O3/1 -> Product5/1
  m.1/1 -> Product5/2
  H2O/1 -> Product4/1
  Normierung auf 1 mol Anteil1/2(Sum) -> Product1/2
  Normierung auf 1 mol Anteil3/2(Sum) -> Product1/1
  Normierung auf 1 mol Anteil3/1(Out1) -> Demux/1
  Normierung auf 1/1 -> Mux5/3
  Mux5/1 -> Switch/3, m.1/1, H2O3/1
  Demux2/3 -> Terminator6/1
  Demux2/2 -> Terminator5/1
  Product1/1 -> Normierung auf 1/1, Display/1, Scope/1, Sum of Elements/1
  Sum of Elements/1 -> Mux5/2
  Demux2/1 -> Mux5/1
  m./1 -> Switch2/1, Product/1, Product4/2
  Molare Masse1/1 -> Product1/4
  Mux4/1 -> Product1/3
  Product2/1 -> Demux1/1
  Add3/1 -> Max/1, Product2/2
  Normierung auf 1 mol Anteil1/1(Out1) -> Product2/1
  mol Anteil/1 -> Mux4/2, Add3/2
  const2/1 -> Add3/1
  Mux3/1 -> Normierung auf 1 mol Anteil1/1(In1)
  Product/1 -> Normierung auf 1 mol Anteil3/1(In1)
  Molare Masse/1 -> Product/3
  x/1 -> Product/2
  "bar -> Pa"/1 -> Mux1/1
  Constant/1 -> Mux1/3
  Mux1/1 -> mol Anteil/1
  Sättigungsdruck [Pa] (Siegel)/1 -> Mux1/2
  Mux2/1 -> Sättigungsdruck [Pa] (Siegel)/1
  Gaseigenschaften/5 -> Terminator2/1
  Gaseigenschaften/4 -> Terminator/1
  Gaseigenschaften/3 -> Terminator3/1
  Gaseigenschaften/1 -> "bar -> Pa"/1
  Konstanten (Siegel)/6(Cf) -> Mux2/7
  Konstanten (Siegel)/5(Ce) -> Mux2/6
  Konstanten (Siegel)/4(Cd) -> Mux2/5
  Konstanten (Siegel)/3(Cc) -> Mux2/4
  Konstanten (Siegel)/2(Cb) -> Mux2/3
  Konstanten (Siegel)/1(Ca) -> Mux2/2
  Gaseigenschaften/2 -> Mux2/1
  Gasvektor in/1 -> Demux3/1, Switch/1, Demux2/1, Demux4/1, H2O/1, Gaseigenschaften/1, x/1, m./1
  Gaseigenschaften/6 -> Terminator7/1
  Add1/1 -> Gain/1, Switch1/2, Switch/2
  Switch/1 -> Switch3/3
  const3/1 -> Switch1/1
  Compare To Constant/1 -> Switch3/2, Switch2/2
  Switch2/1 -> Mux7/2
  Switch1/1 -> Switch2/3
  Demux3/1 -> Mux6/1
  Demux3/3 -> Mux6/3
  const4/1 -> Mux6/2
  Demux3/2 -> Terminator8/1
  Mux6/1 -> Switch3/1
  Switch3/1 -> Gasvektor out/1
  Demux4/1 -> Mux7/1
  Demux4/2 -> Terminator9/1
  Demux4/3 -> Terminator10/1
  x1/1 -> Mux7/3
  Mux7/1 -> waterflow out/1
  Gain/1 -> Switch1/3
  Constant1/1 -> Max/2
  Max/1 -> Product1/5

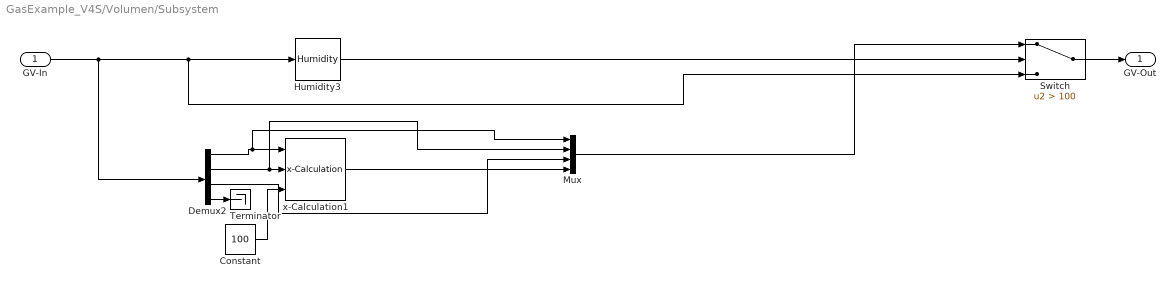
== system GasExample_V4S/Volumen/Subsystem ==
  GV-In : Inport
  Constant : Constant  Value=100
  Demux2 : Demux  Outputs=[1 1 1 4]
  Humidity3 : BibFHDO/Humidity  SystemSampleTime=-1  VariantActivationTime=update diagram  EmptyChoice=off  PassThrough=off  PassThroughVariantControl=(default)  EmptyChoiceVariantControl=(default)  AllowFlexibleInterface=on  Latency=0  AutoFrameSizeCalculation=off
  Mux : Mux  Inputs=[1 1 1 4]
  Switch : Switch  Criteria=u2 > Threshold  Threshold=100  SaturateOnIntegerOverflow=off  InputSameDT=off
  Terminator : Terminator
  x-Calculation1 : BibFHDO/x-Calculation  SystemSampleTime=-1  VariantActivationTime=update diagram  EmptyChoice=off  PassThrough=off  PassThroughVariantControl=(default)  EmptyChoiceVariantControl=(default)  AllowFlexibleInterface=on  Latency=0  AutoFrameSizeCalculation=off
  GV-Out : Outport
  wires:
  Constant/1 -> x-Calculation1/3
  Mux/1 -> Switch/1
  GV-In/1 -> Demux2/1, Humidity3/1, Switch/3
  Humidity3/1 -> Switch/2
  Demux2/2 -> Mux/2, x-Calculation1/2
  Demux2/4 -> Terminator/1
  Demux2/3 -> Mux/3
  Demux2/1 -> Mux/1, x-Calculation1/1
  Switch/1 -> GV-Out/1
  x-Calculation1/1 -> Mux/4

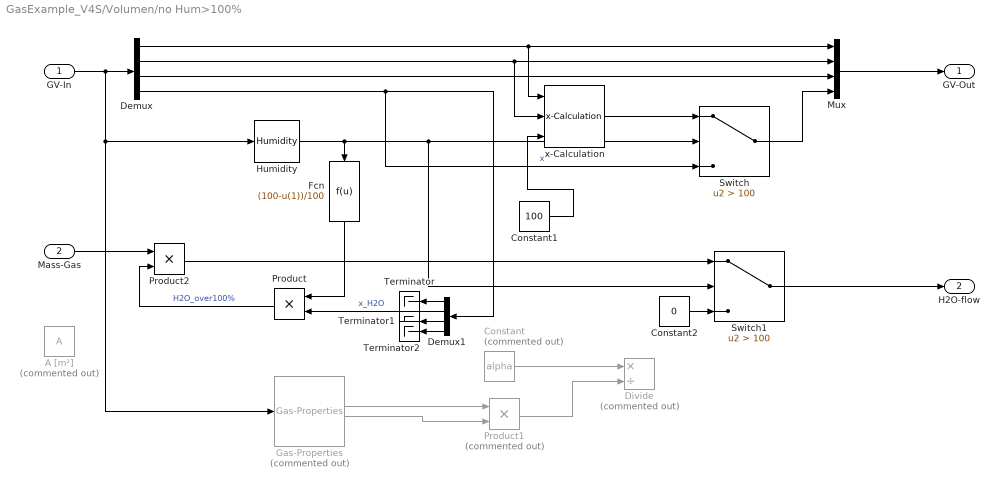
== system GasExample_V4S/Volumen/no Hum>100% ==
  GV-In : Inport
  Mass-Gas : Inport  Port=2
  A [m²] : Constant  Commented=on  Value=A
  Constant : Constant  Commented=on  Value=alpha
  Constant1 : Constant  Value=100
  Constant2 : Constant  Value=0
  Demux : Demux  Outputs=[1 1 1 4]
  Demux1 : Demux
  Divide : Product  Commented=on  Inputs=*/
  Fcn : Fcn  Expr=(100-u(1))/100
  Gas-Properties : BibFHDO/Gas-Properties  Commented=on  SystemSampleTime=-1  VariantActivationTime=update diagram  EmptyChoice=off  PassThrough=off  PassThroughVariantControl=(default)  EmptyChoiceVariantControl=(default)  AllowFlexibleInterface=on  Latency=0  AutoFrameSizeCalculation=off
  Humidity : BibFHDO/Humidity  SystemSampleTime=-1  VariantActivationTime=update diagram  EmptyChoice=off  PassThrough=off  PassThroughVariantControl=(default)  EmptyChoiceVariantControl=(default)  AllowFlexibleInterface=on  Latency=0  AutoFrameSizeCalculation=off
  Mux : Mux
  Product : Product
  Product1 : Product  Commented=on
  Product2 : Product
  Switch : Switch  Criteria=u2 > Threshold  Threshold=100  SaturateOnIntegerOverflow=off  InputSameDT=off
  Switch1 : Switch  Criteria=u2 > Threshold  Threshold=100  SaturateOnIntegerOverflow=off  InputSameDT=off
  Terminator : Terminator
  Terminator1 : Terminator
  Terminator2 : Terminator
  x-Calculation : BibFHDO/x-Calculation  SystemSampleTime=-1  VariantActivationTime=update diagram  EmptyChoice=off  PassThrough=off  PassThroughVariantControl=(default)  EmptyChoiceVariantControl=(default)  AllowFlexibleInterface=on  Latency=0  AutoFrameSizeCalculation=off
  GV-Out : Outport
  H2O-flow : Outport  Port=2
  wires:
  Mass-Gas/1 -> Product2/1
  Product1/1 -> Divide/2
  Constant/1 -> Divide/1
  Gas-Properties/4 -> Product1/2
  Gas-Properties/3 -> Product1/1
  Demux1/3 -> Terminator1/1
  Demux1/4 -> Terminator2/1
  Demux1/1 -> Terminator/1
  Demux1/2 -> Product/2  "x_H2O"
  Fcn/1 -> Product/1
  Product/1 -> Product2/2  "H2O_over100%"
  Humidity/1 -> Switch1/2, Switch/2, Fcn/1
  Mux/1 -> GV-Out/1
  Demux/3 -> Mux/3
  Demux/4 -> Switch/3, Demux1/1  "x"
  Demux/2 -> x-Calculation/2, Mux/2
  Demux/1 -> x-Calculation/1, Mux/1
  GV-In/1 -> Demux/1, Humidity/1, Gas-Properties/1
  Switch/1 -> Mux/4
  x-Calculation/1 -> Switch/1
  Constant1/1 -> x-Calculation/3
  Product2/1 -> Switch1/1
  Switch1/1 -> H2O-flow/1
  Constant2/1 -> Switch1/3

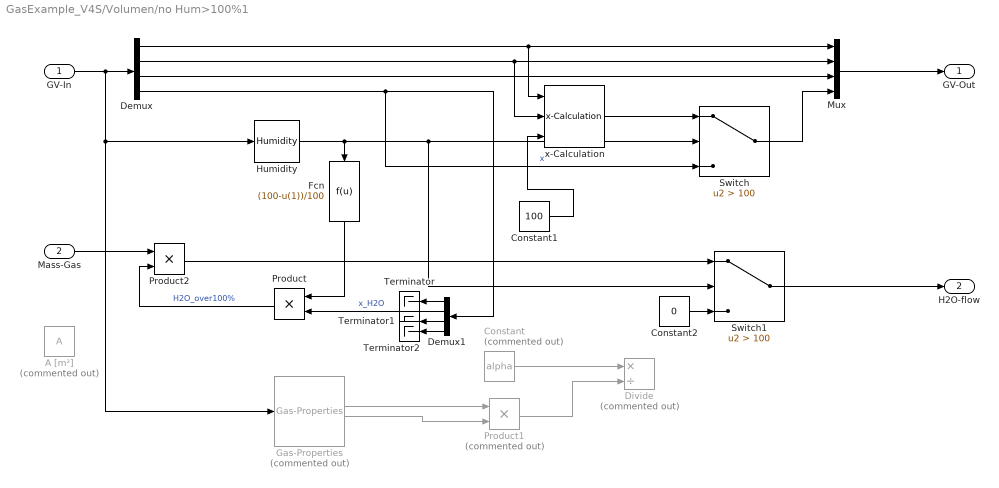
== system GasExample_V4S/Volumen/no Hum>100%1 ==
  GV-In : Inport
  Mass-Gas : Inport  Port=2
  A [m²] : Constant  Commented=on  Value=A
  Constant : Constant  Commented=on  Value=alpha
  Constant1 : Constant  Value=100
  Constant2 : Constant  Value=0
  Demux : Demux  Outputs=[1 1 1 4]
  Demux1 : Demux
  Divide : Product  Commented=on  Inputs=*/
  Fcn : Fcn  Expr=(100-u(1))/100
  Gas-Properties : BibFHDO/Gas-Properties  Commented=on  SystemSampleTime=-1  VariantActivationTime=update diagram  EmptyChoice=off  PassThrough=off  PassThroughVariantControl=(default)  EmptyChoiceVariantControl=(default)  AllowFlexibleInterface=on  Latency=0  AutoFrameSizeCalculation=off
  Humidity : BibFHDO/Humidity  SystemSampleTime=-1  VariantActivationTime=update diagram  EmptyChoice=off  PassThrough=off  PassThroughVariantControl=(default)  EmptyChoiceVariantControl=(default)  AllowFlexibleInterface=on  Latency=0  AutoFrameSizeCalculation=off
  Mux : Mux
  Product : Product
  Product1 : Product  Commented=on
  Product2 : Product
  Switch : Switch  Criteria=u2 > Threshold  Threshold=100  SaturateOnIntegerOverflow=off  InputSameDT=off
  Switch1 : Switch  Criteria=u2 > Threshold  Threshold=100  SaturateOnIntegerOverflow=off  InputSameDT=off
  Terminator : Terminator
  Terminator1 : Terminator
  Terminator2 : Terminator
  x-Calculation : BibFHDO/x-Calculation  SystemSampleTime=-1  VariantActivationTime=update diagram  EmptyChoice=off  PassThrough=off  PassThroughVariantControl=(default)  EmptyChoiceVariantControl=(default)  AllowFlexibleInterface=on  Latency=0  AutoFrameSizeCalculation=off
  GV-Out : Outport
  H2O-flow : Outport  Port=2
  wires:
  Mass-Gas/1 -> Product2/1
  Product1/1 -> Divide/2
  Constant/1 -> Divide/1
  Gas-Properties/4 -> Product1/2
  Gas-Properties/3 -> Product1/1
  Demux1/3 -> Terminator1/1
  Demux1/4 -> Terminator2/1
  Demux1/1 -> Terminator/1
  Demux1/2 -> Product/2  "x_H2O"
  Fcn/1 -> Product/1
  Product/1 -> Product2/2  "H2O_over100%"
  Humidity/1 -> Switch1/2, Switch/2, Fcn/1
  Mux/1 -> GV-Out/1
  Demux/3 -> Mux/3
  Demux/4 -> Switch/3, Demux1/1  "x"
  Demux/2 -> x-Calculation/2, Mux/2
  Demux/1 -> x-Calculation/1, Mux/1
  GV-In/1 -> Demux/1, Humidity/1, Gas-Properties/1
  Switch/1 -> Mux/4
  x-Calculation/1 -> Switch/1
  Constant1/1 -> x-Calculation/3
  Product2/1 -> Switch1/1
  Switch1/1 -> H2O-flow/1
  Constant2/1 -> Switch1/3

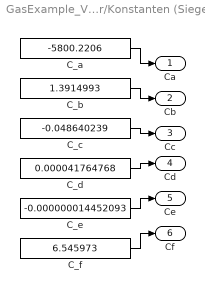
== system GasExample_V4S/Volumen/Befeuchter//Abscheider/Konstanten (Siegel) ==
  C_a : Constant  Value=-5800.2206
  C_b : Constant  Value=1.3914993
  C_c : Constant  Value=-0.048640239
  C_d : Constant  Value=0.000041764768
  C_e : Constant  Value=-0.000000014452093
  C_f : Constant  Value=6.545973
  Ca : Outport
  Cb : Outport  Port=2
  Cc : Outport  Port=3
  Cd : Outport  Port=4
  Ce : Outport  Port=5
  Cf : Outport  Port=6
  wires:
  C_f/1 -> Cf/1
  C_e/1 -> Ce/1
  C_d/1 -> Cd/1
  C_c/1 -> Cc/1
  C_b/1 -> Cb/1
  C_a/1 -> Ca/1

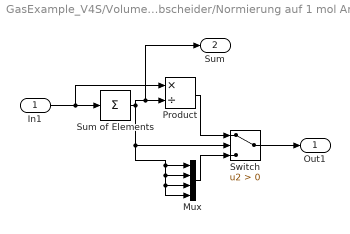
== system GasExample_V4S/Volumen/Befeuchter//Abscheider/Normierung auf 1 mol Anteil1 ==
  In1 : Inport
  Mux : Mux
  Product : Product  Inputs=*/  RndMeth=Zero
  Sum of Elements : Sum  Inputs=+
  Switch : Switch  Criteria=u2 > Threshold  SaturateOnIntegerOverflow=off  InputSameDT=off
  Out1 : Outport
  Sum : Outport  Port=2
  wires:
  In1/1 -> Sum of Elements/1, Product/1
  Sum of Elements/1 -> Switch/2, Mux/4, Mux/3, Mux/2, Mux/1, Product/2, Sum/1
  Product/1 -> Switch/1
  Switch/1 -> Out1/1
  Mux/1 -> Switch/3

== system GasExample_V4S/Volumen/Befeuchter//Abscheider/Normierung auf 1 mol Anteil3 ==
  In1 : Inport
  Mux : Mux
  Product : Product  Inputs=*/  RndMeth=Zero
  Sum of Elements : Sum  Inputs=+
  Switch : Switch  Criteria=u2 > Threshold  SaturateOnIntegerOverflow=off  InputSameDT=off
  Out1 : Outport
  Sum : Outport  Port=2
  wires:
  Mux/1 -> Switch/3
  Switch/1 -> Out1/1
  Product/1 -> Switch/1
  Sum of Elements/1 -> Sum/1, Product/2, Mux/1, Mux/2, Mux/3, Mux/4, Switch/2
  In1/1 -> Product/1, Sum of Elements/1

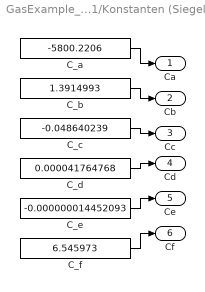
== system GasExample_V4S/Volumen/Befeuchter//Abscheider1/Konstanten (Siegel) ==
  C_a : Constant  Value=-5800.2206
  C_b : Constant  Value=1.3914993
  C_c : Constant  Value=-0.048640239
  C_d : Constant  Value=0.000041764768
  C_e : Constant  Value=-0.000000014452093
  C_f : Constant  Value=6.545973
  Ca : Outport
  Cb : Outport  Port=2
  Cc : Outport  Port=3
  Cd : Outport  Port=4
  Ce : Outport  Port=5
  Cf : Outport  Port=6
  wires:
  C_a/1 -> Ca/1
  C_b/1 -> Cb/1
  C_c/1 -> Cc/1
  C_d/1 -> Cd/1
  C_e/1 -> Ce/1
  C_f/1 -> Cf/1

== system GasExample_V4S/Volumen/Befeuchter//Abscheider1/Normierung auf 1 mol Anteil1 ==
  In1 : Inport
  Mux : Mux
  Product : Product  Inputs=*/  RndMeth=Zero
  Sum of Elements : Sum  Inputs=+
  Switch : Switch  Criteria=u2 > Threshold  SaturateOnIntegerOverflow=off  InputSameDT=off
  Out1 : Outport
  Sum : Outport  Port=2
  wires:
  Mux/1 -> Switch/3
  Switch/1 -> Out1/1
  Product/1 -> Switch/1
  Sum of Elements/1 -> Sum/1, Product/2, Mux/1, Mux/2, Mux/3, Mux/4, Switch/2
  In1/1 -> Product/1, Sum of Elements/1

== system GasExample_V4S/Volumen/Befeuchter//Abscheider1/Normierung auf 1 mol Anteil3 ==
  In1 : Inport
  Mux : Mux
  Product : Product  Inputs=*/  RndMeth=Zero
  Sum of Elements : Sum  Inputs=+
  Switch : Switch  Criteria=u2 > Threshold  SaturateOnIntegerOverflow=off  InputSameDT=off
  Out1 : Outport
  Sum : Outport  Port=2
  wires:
  In1/1 -> Sum of Elements/1, Product/1
  Sum of Elements/1 -> Switch/2, Mux/4, Mux/3, Mux/2, Mux/1, Product/2, Sum/1
  Product/1 -> Switch/1
  Switch/1 -> Out1/1
  Mux/1 -> Switch/3
